simulink subsystem "digitalInputs"  (R2023b)
settings: Solver=VariableStepAuto  StartTime=0.0  StopTime=10.0  RelTol=1e-3
settings Model: Creator=serga  LastModifiedBy=serga
settings OptimizationCC: ReuseModelBlockBuffer=off

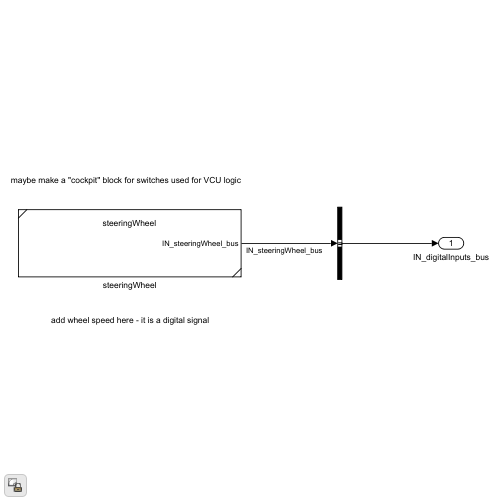
[thumbnail: Simulink's stored preview of the top-level diagram]
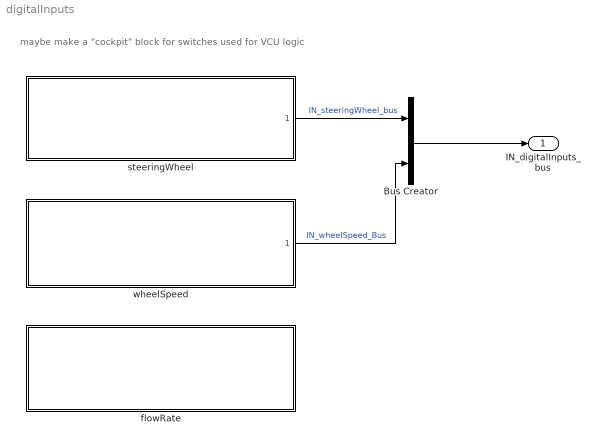
== system digitalInputs ==
  note: maybe make a "cockpit" block for switches used for VCU logic
  Bus Creator : BusCreator  Inputs=2
  flowRate : Subsystem  ReferencedSubsystem=flowRate
  steeringWheel : Subsystem  ReferencedSubsystem=steeringWheel
  wheelSpeed : Subsystem  ReferencedSubsystem=wheelSpeed
  IN_digitalInputs_bus : Outport
  wires:
  Bus Creator/1 -> IN_digitalInputs_bus/1
  steeringWheel/1 -> Bus Creator/1  "IN_steeringWheel_bus"
  wheelSpeed/1 -> Bus Creator/2  "IN_wheelSpeed_Bus"
